simulink model "consigne_couple"  (R2024b)
settings: Solver=FixedStepAuto  StartTime=0.0  StopTime=10.0  FixedStep=Ts  RelTol=1e-3
values from neighbouring files (symbols this model uses):
  G = 4    [main_phi.m]
  Tr = 0.5    [main_phi.m]
  w_wheels = [450 500]    [main_phi.m]
settings Model: Creator=marti  LastModifiedBy=marti

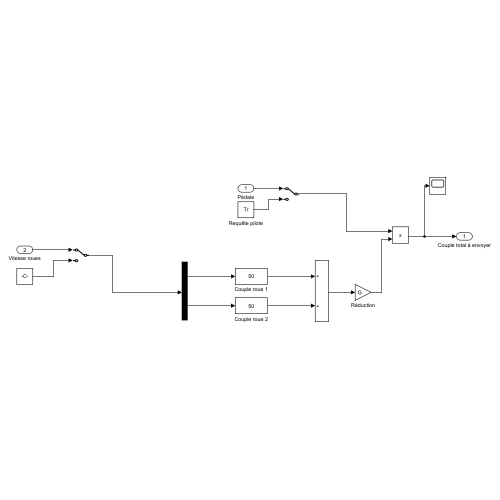
[thumbnail: Simulink's stored preview of the top-level diagram]
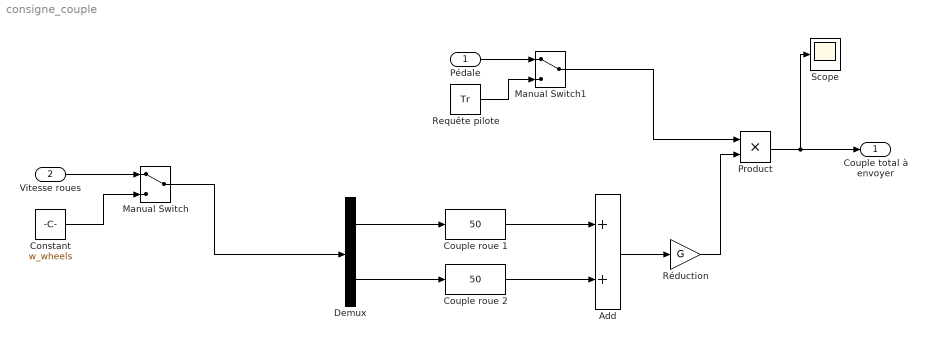
== system consigne_couple ==
  Pédale : Inport
  Vitesse roues : Inport  Port=2  PortDimensions=2
  Add : Sum
  Constant : Constant  Value=w_wheels
  Couple roue 1 : Fcn  Expr=50
  Couple roue 2 : Fcn  Expr=50
  Demux : Demux  Outputs=2
  Manual Switch : ManualSwitch
  Manual Switch1 : ManualSwitch
  Product : Product
  Requête pilote : Constant  Value=Tr
  Réduction : Gain  Gain=G
  Scope : Scope
  Couple total à envoyer : Outport
  wires:
  Add/1 -> Réduction/1
  Réduction/1 -> Product/2
  Pédale/1 -> Manual Switch1/1
  Requête pilote/1 -> Manual Switch1/2
  Manual Switch1/1 -> Product/1
  Product/1 -> Scope/1, Couple total à envoyer/1
  Manual Switch/1 -> Demux/1
  Constant/1 -> Manual Switch/2
  Vitesse roues/1 -> Manual Switch/1
  Demux/1 -> Couple roue 1/1
  Demux/2 -> Couple roue 2/1
  Couple roue 1/1 -> Add/1
  Couple roue 2/1 -> Add/2
